simulink model "scalar_loop_unstable"  (Simulink 8.1)
settings: Solver=ode45  StartTime=0.0  StopTime=10.0  RelTol=1e-3
settings Model: Creator=dejanira  LastModifiedBy=dejanira
settings DataIOCC: SignalLoggingSaveFormat=Dataset
settings OptimizationCC: ExpressionDepthLimit=128
settings DebuggingCC: FcnCallInpInsideContextMsg=EnableAllAsError
settings GRTTargetCC: CombineOutputUpdateFcns=on  GRTInterface=off

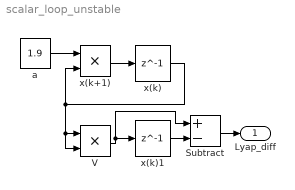
== system scalar_loop_unstable ==
  Subtract : Sum  Inputs=+-
  V : Product
  a : Constant  Value=1.9
  x(k) : Delay  DelayLength=1  SampleTime=0.01
  x(k)1 : Delay  DelayLength=1  InitialCondition=100000  SampleTime=0.01
  x(k+1) : Product
  Lyap_diff : Outport
  wires:
  a/1 -> x(k+1)/1
  x(k+1)/1 -> x(k)/1
  x(k)/1 -> V/2, V/1, x(k+1)/2
  V/1 -> x(k)1/1, Subtract/1
  Subtract/1 -> Lyap_diff/1
  x(k)1/1 -> Subtract/2
